simulink model "model_min_mine"  (R2018a)
settings: Solver=ode45  StartTime=0.0  StopTime=20  RelTol=1e-3
(part 3 of 10)

== system model_min_mine/5 систем підйому/1/7-періодні/7-ми періодна криволінійна ==
  note: затримка на
      |  (t1+t1/)
  note: затримка на
      |  (t1+ t2 + t3)
  note: затримка на
      |  (t1+ t2 +t3 + t4 + t4/)
  (t-2) : Saturate  UpperLimit=3.5  LowerLimit=0
  (t-4) : Saturate  UpperLimit=3.5  LowerLimit=0
  (t-5) : Saturate  LowerLimit=0
  (t1) : Saturate  LowerLimit=0
  Clock1 : Clock
      settings: Decimation=14
  Constant : Constant  Value=2
  Divide : Product  Inputs=/
  Integrator : Integrator
  Product3 : Product  SaturateOnIntegerOverflow=on  OutDataTypeStr=Inherit: Same as first input
  Product5 : Product  SaturateOnIntegerOverflow=on  OutDataTypeStr=Inherit: Same as first input
  Product6 : Product  SaturateOnIntegerOverflow=on  OutDataTypeStr=Inherit: Same as first input
  Scope1 : Scope  NumInputPorts=2
  Scope{3..5,7..9} (6 alike) : Scope
  Scope6 : Scope  NumInputPorts=3
  Subsystem : Subsystem
  Subsystem3 : Subsystem
  Subsystem6 : Subsystem
  Sum1 : Sum  Inputs=|++++  SaturateOnIntegerOverflow=on
  Sum2 : Sum  Inputs=|++++  SaturateOnIntegerOverflow=on
  t1 : DeadZone  LowerValue=0  UpperValue=12  SaturateOnIntegerOverflow=on
  t2 : DeadZone  LowerValue=0  UpperValue=1  SaturateOnIntegerOverflow=on
  t5 : DeadZone  LowerValue=0  UpperValue=8  SaturateOnIntegerOverflow=on
  Допоміжний : Subsystem
  Допоміжний1 : Subsystem
  пакет1 : Subsystem
  пакет2 : Subsystem
  постійні : Subsystem
  Out1 : Outport
  Out2 : Outport  Port=2
  Out3 : Outport  Port=3
  wires:
  t2/1 -> (t-2)/1
  Clock1/1 -> t2/1, t5/1, t1/1, Subsystem6/2(t), Subsystem3/1(t1), (t1)/1, Допоміжний/2(t)
  постійні/5(Out5) -> Subsystem/1(t1)
  постійні/1(Out1) -> Product6/2, Subsystem/3(a1)
  (t-2)/1 -> пакет1/2(t)
  постійні/6(Out6) -> пакет1/1(ti)
  постійні/2(Out2) -> пакет1/3(a)
  t5/1 -> (t-4)/1
  (t-4)/1 -> Допоміжний1/2(t), пакет2/2(t)
  t1/1 -> (t-5)/1
  (t-5)/1 -> Product3/1
  постійні/3(Out3) -> пакет2/3(a)
  постійні/4(Out4) -> Subsystem3/3(a1), Product3/2
  Subsystem6/1(Out1) -> Out1/1, Scope1/1
  Product6/1 -> Sum1/1
  Sum1/1 -> Scope3/1, Out2/1, Scope6/2, Scope1/2, Integrator/1
  Subsystem/1(Out1) -> Sum2/2
  (t1)/1 -> Product6/1, Subsystem/2(t)
  Sum2/1 -> Subsystem6/3(a), Scope7/1
  постійні/9(Out9) -> Subsystem6/1(Сума t)
  Product3/1 -> Sum1/4
  Subsystem3/1(Out1) -> Scope9/1, Sum2/4, Scope6/3
  пакет1/1(Out1) -> Допоміжний/3(a1), Scope8/1
  Допоміжний/1(Out1) -> Sum2/1, Scope5/1
  пакет2/1(Out1) -> Допоміжний1/3(a1)
  Допоміжний1/1(Out1) -> Sum2/3, Scope6/1
  постійні/7(Out7) -> Допоміжний1/1(t1), пакет2/1(ti)
  постійні/8(Out8) -> Subsystem3/2(t)
  постійні/11(Out11) -> Допоміжний/1(t1)
  пакет1/2(Out2) -> Sum1/2
  пакет2/2(Out2) -> Sum1/3
  Integrator/1 -> Product5/2
  Product5/1 -> Scope4/1, Out3/1
  Divide/1 -> Product5/1
  Constant/1 -> Divide/1

== system model_min_mine/5 систем підйому/1/7-періодні/7-ми періодна пр ==
  note: затримка на
      |  (t1+t1/)
  note: затримка на
      |  (t1/+t1+ t2 + t3)
  note: затримка на
      |  (t1+ t2 +t3 + t4 + t4/)
  (t-2) : Saturate  UpperLimit=3.5  LowerLimit=0
  (t-4) : Saturate  UpperLimit=3.5  LowerLimit=0
  (t-5) : Saturate  LowerLimit=0
  (t1) : Saturate  LowerLimit=0
  Clock1 : Clock
      settings: Decimation=17
  Constant : Constant  Value=2
  Divide : Product  Inputs=/
  Integrator : Integrator
  Product{2..6} (5 alike) : Product  SaturateOnIntegerOverflow=on  OutDataTypeStr=Inherit: Same as first input
  Scope1 : Scope  NumInputPorts=2
  Scope{2..3,5,7..9} (6 alike) : Scope
  Scope6 : Scope  NumInputPorts=3
  Subsystem : Subsystem
  Subsystem1 : Subsystem
  Subsystem2 : Subsystem
  Subsystem3 : Subsystem
  Subsystem6 : Subsystem
  Sum1 : Sum  Inputs=|++++  SaturateOnIntegerOverflow=on
  Sum2 : Sum  Inputs=|++++  SaturateOnIntegerOverflow=on
  t1 : DeadZone  LowerValue=0  UpperValue=16  SaturateOnIntegerOverflow=on
  t2 : DeadZone  LowerValue=0  UpperValue=1  SaturateOnIntegerOverflow=on
  t5 : DeadZone  LowerValue=0  UpperValue=12  SaturateOnIntegerOverflow=on
  Допоміжний : Subsystem
  Допоміжний1 : Subsystem
  постійні : Subsystem
  Out1 : Outport
  Out2 : Outport  Port=2
  Out3 : Outport  Port=3
  wires:
  t2/1 -> (t-2)/1
  Clock1/1 -> t2/1, t5/1, t1/1, Subsystem6/2(t), Subsystem3/1(t1), Subsystem2/1(t1), (t1)/1, Допоміжний/2(t)
  постійні/5(Out5) -> Subsystem/1(t1)
  постійні/1(Out1) -> Product6/2, Subsystem/3(a1)
  (t-2)/1 -> Product4/1, Subsystem1/2(t)
  постійні/6(Out6) -> Subsystem1/1(t1)
  постійні/2(Out2) -> Product4/2, Subsystem1/3(a1)
  t5/1 -> (t-4)/1
  (t-4)/1 -> Product2/1, Допоміжний1/2(t)
  t1/1 -> (t-5)/1
  (t-5)/1 -> Product3/1
  постійні/3(Out3) -> Subsystem2/3(a1), Product2/2
  постійні/4(Out4) -> Subsystem3/3(a1), Product3/2
  Subsystem6/1(Out1) -> Out1/1, Scope1/1
  Product4/1 -> Sum1/2
  Product6/1 -> Sum1/1
  Sum1/1 -> Scope3/1, Out2/1, Scope6/2, Scope1/2, Integrator/1
  Subsystem/1(Out1) -> Sum2/2
  (t1)/1 -> Product6/1, Subsystem/2(t)
  Sum2/1 -> Subsystem6/3(a), Scope7/1
  постійні/9(Out9) -> Subsystem6/1(Сума t)
  Product2/1 -> Sum1/3
  Product3/1 -> Sum1/4
  Subsystem3/1(Out1) -> Scope9/1, Sum2/4, Scope6/3
  Subsystem1/1(Out1) -> Допоміжний/3(a1), Scope8/1
  Допоміжний/1(Out1) -> Sum2/1, Scope5/1
  постійні/10(Out10) -> Subsystem2/2(t)
  Subsystem2/1(Out1) -> Допоміжний1/3(a1)
  Допоміжний1/1(Out1) -> Sum2/3, Scope6/1
  постійні/7(Out7) -> Допоміжний1/1(t1)
  постійні/8(Out8) -> Subsystem3/2(t)
  постійні/11(Out11) -> Допоміжний/1(t1)
  Integrator/1 -> Product5/2
  Product5/1 -> Scope2/1, Out3/1
  Divide/1 -> Product5/1
  Constant/1 -> Divide/1

== system model_min_mine/5 систем підйому/2/3-періодні/Криволінійна-3 ==
  (t1) : Saturate  UpperLimit=1.15  LowerLimit=0
  (t1+ t2) : DeadZone  LowerValue=0  UpperValue=3.15  SaturateOnIntegerOverflow=on
  Clock1 : Clock
  Constant : Constant  Value=2
  Constant1 : Constant
  Divide : Product  Inputs=/
  Integrator : Integrator
  Product5 : Product  SaturateOnIntegerOverflow=on  OutDataTypeStr=Inherit: Same as first input
  Scope2 : Scope
  Sum1 : Sum  Inputs=|+-  SaturateOnIntegerOverflow=on
  Sum8 : Sum  Inputs=|++  SaturateOnIntegerOverflow=on
  Sum9 : Sum  Inputs=|++  SaturateOnIntegerOverflow=on
  Switch2 : Switch  Criteria=u2 ~= 0  RndMeth=Zero  SaturateOnIntegerOverflow=on
  T-Загальний час циклу,с : Constant  Value=4.3
  V : Scope
  a : Scope
  t3 : Saturate  UpperLimit=1.15  LowerLimit=0
  Генераці1 : Subsystem  TreatAsAtomicUnit=on
  пакет2 : Subsystem
  пакет3 : Subsystem
  постійні : Subsystem
  Out1 : Outport
  Out2 : Outport  Port=2
  Out3 : Outport  Port=3
  wires:
  (t1+ t2)/1 -> t3/1
  Clock1/1 -> (t1)/1, (t1+ t2)/1, Sum1/2
  T-Загальний час циклу,с/1 -> Sum1/1
  Constant1/1 -> Генераці1/1(In1)
  Sum1/1 -> Генераці1/Trigger
  Генераці1/1(Out1) -> Switch2/2
  пакет3/1(Out1) -> Sum8/2
  пакет3/2(Out2) -> Sum9/2
  пакет2/1(Out1) -> Sum8/1
  Sum8/1 -> Switch2/3, a/1
  Switch2/1 -> Out1/1
  Sum9/1 -> Out2/1, V/1, Integrator/1
  пакет2/2(Out2) -> Sum9/1
  постійні/1(Out1) -> пакет2/3(a)
  постійні/2(Out2) -> пакет3/3(a)
  постійні/4(Out4) -> пакет3/1(ti)
  постійні/3(Out3) -> пакет2/1(ti)
  (t1)/1 -> пакет2/2(t)
  t3/1 -> пакет3/2(t)
  Integrator/1 -> Product5/2
  Product5/1 -> Scope2/1, Out3/1
  Divide/1 -> Product5/1
  Constant/1 -> Divide/1

== system model_min_mine/5 систем підйому/2/3-періодні/Пр ==
  note: (t1+t2)
  (t1) : Saturate  UpperLimit=1.15  LowerLimit=0
  Clock1 : Clock
  Constant : Constant  Value=2
  Constant1 : Constant
  Constant2 : Constant
  Constant5 : Constant
  Divide : Product  Inputs=/
  Integrator : Integrator
  Product2 : Product  SaturateOnIntegerOverflow=on  OutDataTypeStr=Inherit: Same as first input
  Product5 : Product  SaturateOnIntegerOverflow=on  OutDataTypeStr=Inherit: Same as first input
  Product6 : Product  SaturateOnIntegerOverflow=on  OutDataTypeStr=Inherit: Same as first input
  Scope2 : Scope
  Sum1 : Sum  Inputs=|+-  SaturateOnIntegerOverflow=on
  Sum2 : Sum  Inputs=|+-  SaturateOnIntegerOverflow=on
  Sum4 : Sum  Inputs=|+-  SaturateOnIntegerOverflow=on
  Sum8 : Sum  Inputs=|++  SaturateOnIntegerOverflow=on
  Sum9 : Sum  Inputs=|++  SaturateOnIntegerOverflow=on
  Switch1 : Switch  Criteria=u2 ~= 0  RndMeth=Zero  SaturateOnIntegerOverflow=on
  Switch2 : Switch  Criteria=u2 ~= 0  RndMeth=Zero  SaturateOnIntegerOverflow=on
  Switch3 : Switch  Criteria=u2 ~= 0  RndMeth=Zero  SaturateOnIntegerOverflow=on
  T-Загальний час циклу,с : Constant  Value=4.3
  V : Scope
  V1 : Scope
  ogr : Saturate  UpperLimit=100  LowerLimit=0
  t2 : DeadZone  LowerValue=0  UpperValue=3.15  SaturateOnIntegerOverflow=on
  t3 : Saturate  UpperLimit=1.15  LowerLimit=0
  Генераці : Subsystem  TreatAsAtomicUnit=on
  Генераці1 : Subsystem  TreatAsAtomicUnit=on
  Генераці2 : Subsystem  TreatAsAtomicUnit=on
  постійні : Subsystem
  Out1 : Outport
  Out2 : Outport  Port=2
  Out3 : Outport  Port=3
  wires:
  постійні/1(Out1) -> Product6/1, Switch1/3
  t2/1 -> t3/1
  t3/1 -> Product2/2
  Clock1/1 -> (t1)/1, t2/1, Sum2/1, Sum1/2
  (t1)/1 -> Product6/2, Sum4/2
  Product6/1 -> Sum9/1
  постійні/2(Out2) -> Product2/1, Switch2/1
  Product2/1 -> Sum9/2
  Sum9/1 -> ogr/1, V/1, Integrator/1
  Constant5/1 -> Генераці/1(In1)
  Sum4/1 -> Генераці/Trigger
  Генераці/1(Out1) -> Switch1/2
  Switch1/1 -> Sum8/1
  постійні/4(Out4) -> Sum4/1
  Constant1/1 -> Генераці1/1(In1)
  Sum1/1 -> Генераці1/Trigger
  Генераці1/1(Out1) -> Switch2/2
  Switch2/1 -> Sum8/2
  ogr/1 -> Out2/1
  Constant2/1 -> Генераці2/1(In1)
  Генераці2/1(Out1) -> Switch3/2
  Sum2/1 -> Генераці2/Trigger
  Sum8/1 -> Switch3/3
  Switch3/1 -> Out1/1, V1/1
  постійні/5(Out5) -> Sum1/1
  T-Загальний час циклу,с/1 -> Sum2/2
  Integrator/1 -> Product5/2
  Product5/1 -> Scope2/1, Out3/1
  Divide/1 -> Product5/1
  Constant/1 -> Divide/1

== system model_min_mine/5 систем підйому/2/4-періодна /Генераці ==
  In1 : Inport
  Trigger : TriggerPort  TriggerType=either  VariantControl=(inherit)  ShowOutputPort=on
  Out1 : Outport
  wires:
  In1/1 -> Out1/1

== system model_min_mine/5 систем підйому/2/4-періодна /Генераці1 ==
  In1 : Inport
  Trigger : TriggerPort  TriggerType=either  VariantControl=(inherit)  ShowOutputPort=on
  Out1 : Outport
  wires:
  In1/1 -> Out1/1

== system model_min_mine/5 систем підйому/2/4-періодна /Генераці2 ==
  In1 : Inport
  Trigger : TriggerPort  TriggerType=either  VariantControl=(inherit)  ShowOutputPort=on
  Out1 : Outport
  wires:
  In1/1 -> Out1/1

== system model_min_mine/5 систем підйому/2/4-періодна /Генераці3 ==
  In1 : Inport
  Trigger : TriggerPort  TriggerType=either  VariantControl=(inherit)  ShowOutputPort=on
  Out1 : Outport
  wires:
  In1/1 -> Out1/1

== system model_min_mine/5 систем підйому/2/4-періодна /постійні ==
  (t1) : Constant  Value=1.15
  (t3) : Constant  Value=2
  (t4) : Constant
  T : Constant  Value=7.15
  a1 : Constant  Value=0.5
  a3 : Constant  Value=-1
  a4 : Constant  Value=-0.95
  Out1 : Outport
  Out2 : Outport  Port=2
  Out6 : Outport  Port=3
  Out3 : Outport  Port=4
  Out4 : Outport  Port=5
  Out5 : Outport  Port=6
  Out7 : Outport  Port=7
  wires:
  a1/1 -> Out1/1
  a3/1 -> Out2/1
  (t3)/1 -> Out3/1
  (t1)/1 -> Out4/1
  (t4)/1 -> Out5/1
  a4/1 -> Out6/1
  T/1 -> Out7/1

== system model_min_mine/5 систем підйому/2/5-періодні/криво ==
  note: затримка на
      |  (t1)
  note: затримка на
      |  (t1+ t2 + t3)
  note: затримка на
      |  (t1+ t2 +t3 +t4)
  (t-2) : Saturate  UpperLimit=3.5  LowerLimit=0
  (t-4) : Saturate  UpperLimit=3.5  LowerLimit=0
  (t-5) : Saturate  LowerLimit=0
  (t1) : Saturate  LowerLimit=0
  Clock1 : Clock
      settings: Decimation=14
  Constant : Constant  Value=2
  Divide : Product  Inputs=/
  Integrator : Integrator
  Product{2..6} (5 alike) : Product  SaturateOnIntegerOverflow=on  OutDataTypeStr=Inherit: Same as first input
  Scope{1..3,5..7,9} (7 alike) : Scope
  Subsystem : Subsystem
  Subsystem1 : Subsystem
  Subsystem2 : Subsystem
  Subsystem3 : Subsystem
  Subsystem6 : Subsystem
  Sum1 : Sum  Inputs=|++++  SaturateOnIntegerOverflow=on
  Sum2 : Sum  Inputs=|++++  SaturateOnIntegerOverflow=on
  t1 : DeadZone  LowerValue=0  UpperValue=11.5  SaturateOnIntegerOverflow=on
  t2 : DeadZone  LowerValue=0  SaturateOnIntegerOverflow=on
  t5 : DeadZone  LowerValue=0  UpperValue=8  SaturateOnIntegerOverflow=on
  Допоміжний : Subsystem
  Допоміжний1 : Subsystem
  постійні : Subsystem
  Out1 : Outport
  Out2 : Outport  Port=2
  Out3 : Outport  Port=3
  wires:
  t2/1 -> (t-2)/1
  Clock1/1 -> t2/1, t5/1, t1/1, Subsystem6/2(t), Subsystem3/1(t1), Subsystem2/1(t1), (t1)/1
  постійні/5(Out5) -> Subsystem/1(t1)
  постійні/1(Out1) -> Product6/2, Subsystem/3(a1)
  (t-2)/1 -> Product4/1, Subsystem1/2(t)
  постійні/6(Out6) -> Subsystem1/1(t1)
  постійні/2(Out2) -> Product4/2, Subsystem1/3(a1)
  t5/1 -> (t-4)/1
  (t-4)/1 -> Product2/1, Допоміжний1/2(t)
  t1/1 -> (t-5)/1
  (t-5)/1 -> Product3/1
  постійні/3(Out3) -> Subsystem2/3(a1), Product2/2
  постійні/4(Out4) -> Subsystem3/3(a1), Product3/2
  Subsystem6/1(Out1) -> Out1/1, Scope1/1
  Product4/1 -> Sum1/2
  Product6/1 -> Sum1/1
  Sum1/1 -> Scope3/1, Out2/1, Integrator/1
  Subsystem/1(Out1) -> Допоміжний/1(t1), Scope5/1, Sum2/2
  (t1)/1 -> Product6/1, Subsystem/2(t), Допоміжний/2(t)
  Sum2/1 -> Subsystem6/3(a), Scope7/1
  постійні/9(Out9) -> Subsystem6/1(Сума t)
  Product2/1 -> Sum1/3, Scope6/1
  Product3/1 -> Sum1/4
  Subsystem3/1(Out1) -> Scope9/1, Sum2/4
  Subsystem1/1(Out1) -> Допоміжний/3(a1)
  Допоміжний/1(Out1) -> Sum2/1
  постійні/10(Out10) -> Subsystem2/2(t)
  Subsystem2/1(Out1) -> Допоміжний1/3(a1)
  Допоміжний1/1(Out1) -> Sum2/3
  постійні/7(Out7) -> Допоміжний1/1(t1)
  постійні/8(Out8) -> Subsystem3/2(t)
  Integrator/1 -> Product5/2
  Product5/1 -> Scope2/1, Out3/1
  Divide/1 -> Product5/1
  Constant/1 -> Divide/1

== system model_min_mine/5 систем підйому/2/5-періодні/пр ==
  note: затримка на
      |  (t1)
  note: затримка на
      |  (t1+ t2)
  note: затримка на
      |  (t1+ t2 +t3 +t4)
  note: затримка на
      |  (t1+ t2 +t3 +t4 +t5)
  note: затримка на
      |  (t1+ t2 +t3 +t4 +t5 + t6)
  (t-2) : Saturate  UpperLimit=3.5  LowerLimit=0
  (t-3) : Saturate  LowerLimit=0
  (t-5) : Saturate  LowerLimit=0
  (t-6) : Saturate  UpperLimit=3.5  LowerLimit=0
  (t-7) : Saturate  LowerLimit=0
  (t1) : Saturate  LowerLimit=0
  Clock1 : Clock
      settings: Decimation=14
  Constant : Constant  Value=2
  Divide : Product  Inputs=/
  Integrator : Integrator
  Product{1,4..7} (5 alike) : Product  SaturateOnIntegerOverflow=on  OutDataTypeStr=Inherit: Same as first input
  Scope{1..3,5} (4 alike) : Scope
  Subsystem : Subsystem
  Subsystem1 : Subsystem
  Subsystem4 : Subsystem
  Subsystem5 : Subsystem
  Subsystem6 : Subsystem
  Sum1 : Sum  Inputs=|++++++  SaturateOnIntegerOverflow=on
  Sum2 : Sum  Inputs=|++++  SaturateOnIntegerOverflow=on
  Sum3 : Sum  Inputs=-  SaturateOnIntegerOverflow=on
  t1 : DeadZone  LowerValue=0  UpperValue=7.5  SaturateOnIntegerOverflow=on
  t2 : DeadZone  LowerValue=0  SaturateOnIntegerOverflow=on
  t3 : DeadZone  LowerValue=0  UpperValue=8  SaturateOnIntegerOverflow=on
  t4 : DeadZone  LowerValue=0  UpperValue=11.5  SaturateOnIntegerOverflow=on
  t5 : DeadZone  LowerValue=0  UpperValue=4  SaturateOnIntegerOverflow=on
  Допоміжний : Subsystem
  Допоміжний -1 : Subsystem
  Допоміжний -2 : Subsystem
  Допоміжний -3 : Subsystem
  Допоміжний -4 : Subsystem
  пакет1 : Subsystem
  пакет2 : Subsystem
  постійні : Subsystem
  Out1 : Outport
  Out2 : Outport  Port=2
  Out3 : Outport  Port=3
  wires:
  t2/1 -> (t-2)/1
  Clock1/1 -> t2/1, t5/1, t1/1, t3/1, t4/1, Subsystem6/2(t), (t1)/1
  постійні/7(Out7) -> Subsystem/1(t1)
  постійні/1(Out1) -> Product6/2, Subsystem/3(a1)
  (t-2)/1 -> Product4/1, Subsystem1/2(t), Допоміжний -1/2(t)
  постійні/8(Out8) -> Subsystem1/1(t1)
  постійні/2(Out2) -> Product4/2, Subsystem1/3(a1)
  t5/1 -> (t-3)/1
  (t-3)/1 -> пакет1/2(t), Допоміжний -2/2(t)
  t1/1 -> (t-5)/1
  (t-5)/1 -> пакет2/2(t), Допоміжний -3/2(t)
  постійні/9(Out9) -> пакет1/1(ti)
  постійні/11(Out11) -> пакет2/1(ti)
  постійні/3(Out3) -> пакет1/3(a)
  постійні/4(Out4) -> пакет2/3(a)
  t3/1 -> (t-6)/1
  (t-6)/1 -> Product5/1, Subsystem4/2(t), Допоміжний -4/2(t)
  постійні/12(Out12) -> Subsystem4/1(ti)
  постійні/5(Out5) -> Subsystem4/3(a), Product5/2
  t4/1 -> (t-7)/1
  (t-7)/1 -> Subsystem5/2(t), Product7/1
  постійні/13(Out13) -> Subsystem5/1(ti)
  постійні/6(Out6) -> Product7/2, Subsystem5/3(a)
  постійні/10(Out10) -> Subsystem6/1(Сума t)
  Subsystem6/1(Out1) -> Out1/1, Scope1/1
  Product4/1 -> Sum1/2
  Product6/1 -> Sum1/1
  пакет1/2(Out2) -> Sum1/3
  пакет2/2(Out2) -> Sum1/4
  Product5/1 -> Sum1/5
  Product7/1 -> Sum1/6
  Sum1/1 -> Scope3/1, Out2/1, Integrator/1
  Subsystem/1(Out1) -> Допоміжний/1(t1), Sum2/2, Scope5/1
  (t1)/1 -> Product6/1, Subsystem/2(t), Допоміжний/2(t)
  Subsystem1/1(Out1) -> Допоміжний/3(a1)
  Допоміжний/1(Out1) -> Допоміжний -1/1(t1)
  пакет1/1(Out1) -> Допоміжний -1/3(a1)
  Допоміжний -1/1(Out1) -> Допоміжний -2/1(t1), Sum2/1
  пакет2/1(Out1) -> Допоміжний -2/3(a1)
  Допоміжний -2/1(Out1) -> Допоміжний -3/1(t1), Sum2/3
  Subsystem4/1(Out1) -> Допоміжний -3/3(a1)
  Допоміжний -3/1(Out1) -> Допоміжний -4/1(t1)
  Subsystem5/1(Out1) -> Допоміжний -4/3(a1)
  Sum2/1 -> Subsystem6/3(a)
  Допоміжний -4/1(Out1) -> Sum3/1
  Sum3/1 -> Sum2/4
  Integrator/1 -> Product1/2
  Product1/1 -> Scope2/1, Out3/1
  Divide/1 -> Product1/1
  Constant/1 -> Divide/1

== system model_min_mine/5 систем підйому/2/6-періодні/6-ти періодна криволінійна ==
  note: затримка на
      |  (t1)
  note: затримка на
      |  (t1+ t2 + t3)
  note: затримка на
      |  (t1+ t2 +t3 +t4 +t4/)
  (t-2) : Saturate  UpperLimit=3.5  LowerLimit=0
  (t-4) : Saturate  UpperLimit=3.5  LowerLimit=0
  (t-5) : Saturate  LowerLimit=0
  (t1) : Saturate  LowerLimit=0
  Clock1 : Clock
      settings: Decimation=14
  Constant : Constant  Value=2
  Divide : Product  Inputs=/
  Integrator : Integrator
  Product3 : Product  SaturateOnIntegerOverflow=on  OutDataTypeStr=Inherit: Same as first input
  Product5 : Product  SaturateOnIntegerOverflow=on  OutDataTypeStr=Inherit: Same as first input
  Product6 : Product  SaturateOnIntegerOverflow=on  OutDataTypeStr=Inherit: Same as first input
  Scope{1..3,5,7,9} (6 alike) : Scope
  Scope6 : Scope  NumInputPorts=3
  Subsystem : Subsystem
  Subsystem3 : Subsystem
  Subsystem6 : Subsystem
  Sum1 : Sum  Inputs=|++++  SaturateOnIntegerOverflow=on
  Sum2 : Sum  Inputs=|++++  SaturateOnIntegerOverflow=on
  t1 : DeadZone  LowerValue=0  UpperValue=12  SaturateOnIntegerOverflow=on
  t2 : DeadZone  LowerValue=0  SaturateOnIntegerOverflow=on
  t5 : DeadZone  LowerValue=0  UpperValue=8  SaturateOnIntegerOverflow=on
  Допоміжний : Subsystem
  Допоміжний1 : Subsystem
  пакет1 : Subsystem
  пакет2 : Subsystem
  постійні : Subsystem
  Out1 : Outport
  Out2 : Outport  Port=2
  Out3 : Outport  Port=3
  wires:
  t2/1 -> (t-2)/1
  Clock1/1 -> (t1)/1, t2/1, t5/1, t1/1, Subsystem6/2(t), Subsystem3/1(t1)
  постійні/5(Out5) -> Subsystem/1(t1)
  постійні/1(Out1) -> Product6/2, Subsystem/3(a1)
  (t-2)/1 -> пакет1/2(t)
  постійні/6(Out6) -> пакет1/1(ti)
  постійні/2(Out2) -> пакет1/3(a)
  t5/1 -> (t-4)/1
  (t-4)/1 -> Допоміжний1/2(t), пакет2/2(t)
  t1/1 -> (t-5)/1
  (t-5)/1 -> Product3/1
  постійні/3(Out3) -> пакет2/3(a)
  постійні/4(Out4) -> Subsystem3/3(a1), Product3/2
  Subsystem6/1(Out1) -> Out1/1, Scope1/1
  Product6/1 -> Sum1/1
  Sum1/1 -> Scope3/1, Out2/1, Scope6/2, Integrator/1
  Subsystem/1(Out1) -> Допоміжний/1(t1), Scope5/1, Sum2/2
  (t1)/1 -> Product6/1, Subsystem/2(t), Допоміжний/2(t)
  Sum2/1 -> Subsystem6/3(a), Scope7/1
  постійні/9(Out9) -> Subsystem6/1(Сума t)
  Product3/1 -> Sum1/4
  Subsystem3/1(Out1) -> Scope9/1, Sum2/4, Scope6/3
  пакет1/1(Out1) -> Допоміжний/3(a1)
  Допоміжний/1(Out1) -> Sum2/1
  пакет2/1(Out1) -> Допоміжний1/3(a1)
  Допоміжний1/1(Out1) -> Sum2/3, Scope6/1
  постійні/7(Out7) -> Допоміжний1/1(t1), пакет2/1(ti)
  постійні/8(Out8) -> Subsystem3/2(t)
  пакет1/2(Out2) -> Sum1/2
  пакет2/2(Out2) -> Sum1/3
  Integrator/1 -> Product5/2
  Product5/1 -> Scope2/1, Out3/1
  Divide/1 -> Product5/1
  Constant/1 -> Divide/1

== system model_min_mine/5 систем підйому/2/6-періодні/6-ти періодна пр ==
  note: затримка на
      |  (t1)
  note: затримка на
      |  (t1+ t2 + t3)
  note: затримка на
      |  (t1+ t2 +t3 +t4 +t4/)
  (t-2) : Saturate  UpperLimit=3.5  LowerLimit=0
  (t-4) : Saturate  UpperLimit=3.5  LowerLimit=0
  (t-5) : Saturate  LowerLimit=0
  (t1) : Saturate  LowerLimit=0
  Clock1 : Clock
      settings: Decimation=14
  Constant : Constant  Value=2
  Divide : Product  Inputs=/
  Integrator : Integrator
  Product{2..6} (5 alike) : Product  SaturateOnIntegerOverflow=on  OutDataTypeStr=Inherit: Same as first input
  Scope{1..3,5,7,9} (6 alike) : Scope
  Scope6 : Scope  NumInputPorts=3
  Subsystem : Subsystem
  Subsystem1 : Subsystem
  Subsystem2 : Subsystem
  Subsystem3 : Subsystem
  Subsystem6 : Subsystem
  Sum1 : Sum  Inputs=|++++  SaturateOnIntegerOverflow=on
  Sum2 : Sum  Inputs=|++++  SaturateOnIntegerOverflow=on
  t1 : DeadZone  LowerValue=0  UpperValue=12  SaturateOnIntegerOverflow=on
  t2 : DeadZone  LowerValue=0  SaturateOnIntegerOverflow=on
  t5 : DeadZone  LowerValue=0  UpperValue=8  SaturateOnIntegerOverflow=on
  Допоміжний : Subsystem
  Допоміжний1 : Subsystem
  постійні : Subsystem
  Out1 : Outport
  Out2 : Outport  Port=2
  Out3 : Outport  Port=3
  wires:
  t2/1 -> (t-2)/1
  Clock1/1 -> t2/1, t5/1, t1/1, Subsystem6/2(t), Subsystem3/1(t1), Subsystem2/1(t1), (t1)/1
  постійні/5(Out5) -> Subsystem/1(t1)
  постійні/1(Out1) -> Product6/2, Subsystem/3(a1)
  (t-2)/1 -> Product4/1, Subsystem1/2(t)
  постійні/6(Out6) -> Subsystem1/1(t1)
  постійні/2(Out2) -> Product4/2, Subsystem1/3(a1)
  t5/1 -> (t-4)/1
  (t-4)/1 -> Product2/1, Допоміжний1/2(t)
  t1/1 -> (t-5)/1
  (t-5)/1 -> Product3/1
  постійні/3(Out3) -> Subsystem2/3(a1), Product2/2
  постійні/4(Out4) -> Subsystem3/3(a1), Product3/2
  Subsystem6/1(Out1) -> Out1/1, Scope1/1
  Product4/1 -> Sum1/2
  Product6/1 -> Sum1/1
  Sum1/1 -> Scope3/1, Out2/1, Scope6/2, Integrator/1
  Subsystem/1(Out1) -> Допоміжний/1(t1), Scope5/1, Sum2/2
  (t1)/1 -> Product6/1, Subsystem/2(t), Допоміжний/2(t)
  Sum2/1 -> Subsystem6/3(a), Scope7/1
  постійні/9(Out9) -> Subsystem6/1(Сума t)
  Product2/1 -> Sum1/3
  Product3/1 -> Sum1/4
  Subsystem3/1(Out1) -> Scope9/1, Sum2/4, Scope6/3
  Subsystem1/1(Out1) -> Допоміжний/3(a1)
  Допоміжний/1(Out1) -> Sum2/1
  постійні/10(Out10) -> Subsystem2/2(t)
  Subsystem2/1(Out1) -> Допоміжний1/3(a1)
  Допоміжний1/1(Out1) -> Sum2/3, Scope6/1
  постійні/7(Out7) -> Допоміжний1/1(t1)
  постійні/8(Out8) -> Subsystem3/2(t)
  Integrator/1 -> Product5/2
  Product5/1 -> Scope2/1, Out3/1
  Divide/1 -> Product5/1
  Constant/1 -> Divide/1

== system model_min_mine/5 систем підйому/2/7-періодні/7-ми періодна криволінійна ==
  note: затримка на
      |  (t1+t1/)
  note: затримка на
      |  (t1+ t2 + t3)
  note: затримка на
      |  (t1+ t2 +t3 + t4 + t4/)
  (t-2) : Saturate  UpperLimit=3.5  LowerLimit=0
  (t-4) : Saturate  UpperLimit=3.5  LowerLimit=0
  (t-5) : Saturate  LowerLimit=0
  (t1) : Saturate  LowerLimit=0
  Clock1 : Clock
      settings: Decimation=14
  Constant : Constant  Value=2
  Divide : Product  Inputs=/
  Integrator : Integrator
  Product3 : Product  SaturateOnIntegerOverflow=on  OutDataTypeStr=Inherit: Same as first input
  Product5 : Product  SaturateOnIntegerOverflow=on  OutDataTypeStr=Inherit: Same as first input
  Product6 : Product  SaturateOnIntegerOverflow=on  OutDataTypeStr=Inherit: Same as first input
  Scope1 : Scope  NumInputPorts=2
  Scope{3..5,7..9} (6 alike) : Scope
  Scope6 : Scope  NumInputPorts=3
  Subsystem : Subsystem
  Subsystem3 : Subsystem
  Subsystem6 : Subsystem
  Sum1 : Sum  Inputs=|++++  SaturateOnIntegerOverflow=on
  Sum2 : Sum  Inputs=|++++  SaturateOnIntegerOverflow=on
  t1 : DeadZone  LowerValue=0  UpperValue=12  SaturateOnIntegerOverflow=on
  t2 : DeadZone  LowerValue=0  UpperValue=1  SaturateOnIntegerOverflow=on
  t5 : DeadZone  LowerValue=0  UpperValue=8  SaturateOnIntegerOverflow=on
  Допоміжний : Subsystem
  Допоміжний1 : Subsystem
  пакет1 : Subsystem
  пакет2 : Subsystem
  постійні : Subsystem
  Out1 : Outport
  Out2 : Outport  Port=2
  Out3 : Outport  Port=3
  wires:
  t2/1 -> (t-2)/1
  Clock1/1 -> t2/1, t5/1, t1/1, Subsystem6/2(t), Subsystem3/1(t1), (t1)/1, Допоміжний/2(t)
  постійні/5(Out5) -> Subsystem/1(t1)
  постійні/1(Out1) -> Product6/2, Subsystem/3(a1)
  (t-2)/1 -> пакет1/2(t)
  постійні/6(Out6) -> пакет1/1(ti)
  постійні/2(Out2) -> пакет1/3(a)
  t5/1 -> (t-4)/1
  (t-4)/1 -> Допоміжний1/2(t), пакет2/2(t)
  t1/1 -> (t-5)/1
  (t-5)/1 -> Product3/1
  постійні/3(Out3) -> пакет2/3(a)
  постійні/4(Out4) -> Subsystem3/3(a1), Product3/2
  Subsystem6/1(Out1) -> Out1/1, Scope1/1
  Product6/1 -> Sum1/1
  Sum1/1 -> Scope3/1, Out2/1, Scope6/2, Scope1/2, Integrator/1
  Subsystem/1(Out1) -> Sum2/2
  (t1)/1 -> Product6/1, Subsystem/2(t)
  Sum2/1 -> Subsystem6/3(a), Scope7/1
  постійні/9(Out9) -> Subsystem6/1(Сума t)
  Product3/1 -> Sum1/4
  Subsystem3/1(Out1) -> Scope9/1, Sum2/4, Scope6/3
  пакет1/1(Out1) -> Допоміжний/3(a1), Scope8/1
  Допоміжний/1(Out1) -> Sum2/1, Scope5/1
  пакет2/1(Out1) -> Допоміжний1/3(a1)
  Допоміжний1/1(Out1) -> Sum2/3, Scope6/1
  постійні/7(Out7) -> Допоміжний1/1(t1), пакет2/1(ti)
  постійні/8(Out8) -> Subsystem3/2(t)
  постійні/11(Out11) -> Допоміжний/1(t1)
  пакет1/2(Out2) -> Sum1/2
  пакет2/2(Out2) -> Sum1/3
  Integrator/1 -> Product5/2
  Product5/1 -> Scope4/1, Out3/1
  Divide/1 -> Product5/1
  Constant/1 -> Divide/1

== system model_min_mine/5 систем підйому/2/7-періодні/7-ми періодна пр ==
  note: затримка на
      |  (t1+t1/)
  note: затримка на
      |  (t1/+t1+ t2 + t3)
  note: затримка на
      |  (t1+ t2 +t3 + t4 + t4/)
  (t-2) : Saturate  UpperLimit=3.5  LowerLimit=0
  (t-4) : Saturate  UpperLimit=3.5  LowerLimit=0
  (t-5) : Saturate  LowerLimit=0
  (t1) : Saturate  LowerLimit=0
  Clock1 : Clock
      settings: Decimation=17
  Constant : Constant  Value=2
  Divide : Product  Inputs=/
  Integrator : Integrator
  Product{2..6} (5 alike) : Product  SaturateOnIntegerOverflow=on  OutDataTypeStr=Inherit: Same as first input
  Scope1 : Scope  NumInputPorts=2
  Scope{2..3,5,7..9} (6 alike) : Scope
  Scope6 : Scope  NumInputPorts=3
  Subsystem : Subsystem
  Subsystem1 : Subsystem
  Subsystem2 : Subsystem
  Subsystem3 : Subsystem
  Subsystem6 : Subsystem
  Sum1 : Sum  Inputs=|++++  SaturateOnIntegerOverflow=on
  Sum2 : Sum  Inputs=|++++  SaturateOnIntegerOverflow=on
  t1 : DeadZone  LowerValue=0  UpperValue=16  SaturateOnIntegerOverflow=on
  t2 : DeadZone  LowerValue=0  UpperValue=1  SaturateOnIntegerOverflow=on
  t5 : DeadZone  LowerValue=0  UpperValue=12  SaturateOnIntegerOverflow=on
  Допоміжний : Subsystem
  Допоміжний1 : Subsystem
  постійні : Subsystem
  Out1 : Outport
  Out2 : Outport  Port=2
  Out3 : Outport  Port=3
  wires:
  t2/1 -> (t-2)/1
  Clock1/1 -> t2/1, t5/1, t1/1, Subsystem6/2(t), Subsystem3/1(t1), Subsystem2/1(t1), (t1)/1, Допоміжний/2(t)
  постійні/5(Out5) -> Subsystem/1(t1)
  постійні/1(Out1) -> Product6/2, Subsystem/3(a1)
  (t-2)/1 -> Product4/1, Subsystem1/2(t)
  постійні/6(Out6) -> Subsystem1/1(t1)
  постійні/2(Out2) -> Product4/2, Subsystem1/3(a1)
  t5/1 -> (t-4)/1
  (t-4)/1 -> Product2/1, Допоміжний1/2(t)
  t1/1 -> (t-5)/1
  (t-5)/1 -> Product3/1
  постійні/3(Out3) -> Subsystem2/3(a1), Product2/2
  постійні/4(Out4) -> Subsystem3/3(a1), Product3/2
  Subsystem6/1(Out1) -> Out1/1, Scope1/1
  Product4/1 -> Sum1/2
  Product6/1 -> Sum1/1
  Sum1/1 -> Scope3/1, Out2/1, Scope6/2, Scope1/2, Integrator/1
  Subsystem/1(Out1) -> Sum2/2
  (t1)/1 -> Product6/1, Subsystem/2(t)
  Sum2/1 -> Subsystem6/3(a), Scope7/1
  постійні/9(Out9) -> Subsystem6/1(Сума t)
  Product2/1 -> Sum1/3
  Product3/1 -> Sum1/4
  Subsystem3/1(Out1) -> Scope9/1, Sum2/4, Scope6/3
  Subsystem1/1(Out1) -> Допоміжний/3(a1), Scope8/1
  Допоміжний/1(Out1) -> Sum2/1, Scope5/1
  постійні/10(Out10) -> Subsystem2/2(t)
  Subsystem2/1(Out1) -> Допоміжний1/3(a1)
  Допоміжний1/1(Out1) -> Sum2/3, Scope6/1
  постійні/7(Out7) -> Допоміжний1/1(t1)
  постійні/8(Out8) -> Subsystem3/2(t)
  постійні/11(Out11) -> Допоміжний/1(t1)
  Integrator/1 -> Product5/2
  Product5/1 -> Scope2/1, Out3/1
  Divide/1 -> Product5/1
  Constant/1 -> Divide/1

== system model_min_mine/5 систем підйому/3/3-періодні/Криволінійна-3 ==
  (t1) : Saturate  UpperLimit=1.15  LowerLimit=0
  (t1+ t2) : DeadZone  LowerValue=0  UpperValue=3.15  SaturateOnIntegerOverflow=on
  Clock1 : Clock
  Constant : Constant  Value=2
  Constant1 : Constant
  Divide : Product  Inputs=/
  Integrator : Integrator
  Product5 : Product  SaturateOnIntegerOverflow=on  OutDataTypeStr=Inherit: Same as first input
  Scope2 : Scope
  Sum1 : Sum  Inputs=|+-  SaturateOnIntegerOverflow=on
  Sum8 : Sum  Inputs=|++  SaturateOnIntegerOverflow=on
  Sum9 : Sum  Inputs=|++  SaturateOnIntegerOverflow=on
  Switch2 : Switch  Criteria=u2 ~= 0  RndMeth=Zero  SaturateOnIntegerOverflow=on
  T-Загальний час циклу,с : Constant  Value=4.3
  V : Scope
  a : Scope
  t3 : Saturate  UpperLimit=1.15  LowerLimit=0
  Генераці1 : Subsystem  TreatAsAtomicUnit=on
  пакет2 : Subsystem
  пакет3 : Subsystem
  постійні : Subsystem
  Out1 : Outport
  Out2 : Outport  Port=2
  Out3 : Outport  Port=3
  wires:
  (t1+ t2)/1 -> t3/1
  Clock1/1 -> (t1)/1, (t1+ t2)/1, Sum1/2
  T-Загальний час циклу,с/1 -> Sum1/1
  Constant1/1 -> Генераці1/1(In1)
  Sum1/1 -> Генераці1/Trigger
  Генераці1/1(Out1) -> Switch2/2
  пакет3/1(Out1) -> Sum8/2
  пакет3/2(Out2) -> Sum9/2
  пакет2/1(Out1) -> Sum8/1
  Sum8/1 -> Switch2/3, a/1
  Switch2/1 -> Out1/1
  Sum9/1 -> Out2/1, V/1, Integrator/1
  пакет2/2(Out2) -> Sum9/1
  постійні/1(Out1) -> пакет2/3(a)
  постійні/2(Out2) -> пакет3/3(a)
  постійні/4(Out4) -> пакет3/1(ti)
  постійні/3(Out3) -> пакет2/1(ti)
  (t1)/1 -> пакет2/2(t)
  t3/1 -> пакет3/2(t)
  Integrator/1 -> Product5/2
  Product5/1 -> Scope2/1, Out3/1
  Divide/1 -> Product5/1
  Constant/1 -> Divide/1

== system model_min_mine/5 систем підйому/3/3-періодні/Пр ==
  note: (t1+t2)
  (t1) : Saturate  UpperLimit=1.15  LowerLimit=0
  Clock1 : Clock
  Constant : Constant  Value=2
  Constant1 : Constant
  Constant2 : Constant
  Constant5 : Constant
  Divide : Product  Inputs=/
  Integrator : Integrator
  Product2 : Product  SaturateOnIntegerOverflow=on  OutDataTypeStr=Inherit: Same as first input
  Product5 : Product  SaturateOnIntegerOverflow=on  OutDataTypeStr=Inherit: Same as first input
  Product6 : Product  SaturateOnIntegerOverflow=on  OutDataTypeStr=Inherit: Same as first input
  Scope2 : Scope
  Sum1 : Sum  Inputs=|+-  SaturateOnIntegerOverflow=on
  Sum2 : Sum  Inputs=|+-  SaturateOnIntegerOverflow=on
  Sum4 : Sum  Inputs=|+-  SaturateOnIntegerOverflow=on
  Sum8 : Sum  Inputs=|++  SaturateOnIntegerOverflow=on
  Sum9 : Sum  Inputs=|++  SaturateOnIntegerOverflow=on
  Switch1 : Switch  Criteria=u2 ~= 0  RndMeth=Zero  SaturateOnIntegerOverflow=on
  Switch2 : Switch  Criteria=u2 ~= 0  RndMeth=Zero  SaturateOnIntegerOverflow=on
  Switch3 : Switch  Criteria=u2 ~= 0  RndMeth=Zero  SaturateOnIntegerOverflow=on
  T-Загальний час циклу,с : Constant  Value=4.3
  V : Scope
  V1 : Scope
  ogr : Saturate  UpperLimit=100  LowerLimit=0
  t2 : DeadZone  LowerValue=0  UpperValue=3.15  SaturateOnIntegerOverflow=on
  t3 : Saturate  UpperLimit=1.15  LowerLimit=0
  Генераці : Subsystem  TreatAsAtomicUnit=on
  Генераці1 : Subsystem  TreatAsAtomicUnit=on
  Генераці2 : Subsystem  TreatAsAtomicUnit=on
  постійні : Subsystem
  Out1 : Outport
  Out2 : Outport  Port=2
  Out3 : Outport  Port=3
  wires:
  постійні/1(Out1) -> Product6/1, Switch1/3
  t2/1 -> t3/1
  t3/1 -> Product2/2
  Clock1/1 -> (t1)/1, t2/1, Sum2/1, Sum1/2
  (t1)/1 -> Product6/2, Sum4/2
  Product6/1 -> Sum9/1
  постійні/2(Out2) -> Product2/1, Switch2/1
  Product2/1 -> Sum9/2
  Sum9/1 -> ogr/1, V/1, Integrator/1
  Constant5/1 -> Генераці/1(In1)
  Sum4/1 -> Генераці/Trigger
  Генераці/1(Out1) -> Switch1/2
  Switch1/1 -> Sum8/1
  постійні/4(Out4) -> Sum4/1
  Constant1/1 -> Генераці1/1(In1)
  Sum1/1 -> Генераці1/Trigger
  Генераці1/1(Out1) -> Switch2/2
  Switch2/1 -> Sum8/2
  ogr/1 -> Out2/1
  Constant2/1 -> Генераці2/1(In1)
  Генераці2/1(Out1) -> Switch3/2
  Sum2/1 -> Генераці2/Trigger
  Sum8/1 -> Switch3/3
  Switch3/1 -> Out1/1, V1/1
  постійні/5(Out5) -> Sum1/1
  T-Загальний час циклу,с/1 -> Sum2/2
  Integrator/1 -> Product5/2
  Product5/1 -> Scope2/1, Out3/1
  Divide/1 -> Product5/1
  Constant/1 -> Divide/1

== system model_min_mine/5 систем підйому/3/4-періодна /Генераці ==
  In1 : Inport
  Trigger : TriggerPort  TriggerType=either  VariantControl=(inherit)  ShowOutputPort=on
  Out1 : Outport
  wires:
  In1/1 -> Out1/1

== system model_min_mine/5 систем підйому/3/4-періодна /Генераці1 ==
  In1 : Inport
  Trigger : TriggerPort  TriggerType=either  VariantControl=(inherit)  ShowOutputPort=on
  Out1 : Outport
  wires:
  In1/1 -> Out1/1

== system model_min_mine/5 систем підйому/3/4-періодна /Генераці2 ==
  In1 : Inport
  Trigger : TriggerPort  TriggerType=either  VariantControl=(inherit)  ShowOutputPort=on
  Out1 : Outport
  wires:
  In1/1 -> Out1/1

== system model_min_mine/5 систем підйому/3/4-періодна /Генераці3 ==
  In1 : Inport
  Trigger : TriggerPort  TriggerType=either  VariantControl=(inherit)  ShowOutputPort=on
  Out1 : Outport
  wires:
  In1/1 -> Out1/1

== system model_min_mine/5 систем підйому/3/4-періодна /постійні ==
  (t1) : Constant  Value=1.15
  (t3) : Constant  Value=2
  (t4) : Constant
  T : Constant  Value=7.15
  a1 : Constant  Value=0.5
  a3 : Constant  Value=-1
  a4 : Constant  Value=-0.95
  Out1 : Outport
  Out2 : Outport  Port=2
  Out6 : Outport  Port=3
  Out3 : Outport  Port=4
  Out4 : Outport  Port=5
  Out5 : Outport  Port=6
  Out7 : Outport  Port=7
  wires:
  a1/1 -> Out1/1
  a3/1 -> Out2/1
  (t3)/1 -> Out3/1
  (t1)/1 -> Out4/1
  (t4)/1 -> Out5/1
  a4/1 -> Out6/1
  T/1 -> Out7/1

== system model_min_mine/5 систем підйому/3/5-періодні/криво ==
  note: затримка на
      |  (t1)
  note: затримка на
      |  (t1+ t2 + t3)
  note: затримка на
      |  (t1+ t2 +t3 +t4)
  (t-2) : Saturate  UpperLimit=3.5  LowerLimit=0
  (t-4) : Saturate  UpperLimit=3.5  LowerLimit=0
  (t-5) : Saturate  LowerLimit=0
  (t1) : Saturate  LowerLimit=0
  Clock1 : Clock
      settings: Decimation=14
  Constant : Constant  Value=2
  Divide : Product  Inputs=/
  Integrator : Integrator
  Product{2..6} (5 alike) : Product  SaturateOnIntegerOverflow=on  OutDataTypeStr=Inherit: Same as first input
  Scope{1..3,5..7,9} (7 alike) : Scope
  Subsystem : Subsystem
  Subsystem1 : Subsystem
  Subsystem2 : Subsystem
  Subsystem3 : Subsystem
  Subsystem6 : Subsystem
  Sum1 : Sum  Inputs=|++++  SaturateOnIntegerOverflow=on
  Sum2 : Sum  Inputs=|++++  SaturateOnIntegerOverflow=on
  t1 : DeadZone  LowerValue=0  UpperValue=11.5  SaturateOnIntegerOverflow=on
  t2 : DeadZone  LowerValue=0  SaturateOnIntegerOverflow=on
  t5 : DeadZone  LowerValue=0  UpperValue=8  SaturateOnIntegerOverflow=on
  Допоміжний : Subsystem
  Допоміжний1 : Subsystem
  постійні : Subsystem
  Out1 : Outport
  Out2 : Outport  Port=2
  Out3 : Outport  Port=3
  wires:
  t2/1 -> (t-2)/1
  Clock1/1 -> t2/1, t5/1, t1/1, Subsystem6/2(t), Subsystem3/1(t1), Subsystem2/1(t1), (t1)/1
  постійні/5(Out5) -> Subsystem/1(t1)
  постійні/1(Out1) -> Product6/2, Subsystem/3(a1)
  (t-2)/1 -> Product4/1, Subsystem1/2(t)
  постійні/6(Out6) -> Subsystem1/1(t1)
  постійні/2(Out2) -> Product4/2, Subsystem1/3(a1)
  t5/1 -> (t-4)/1
  (t-4)/1 -> Product2/1, Допоміжний1/2(t)
  t1/1 -> (t-5)/1
  (t-5)/1 -> Product3/1
  постійні/3(Out3) -> Subsystem2/3(a1), Product2/2
  постійні/4(Out4) -> Subsystem3/3(a1), Product3/2
  Subsystem6/1(Out1) -> Out1/1, Scope1/1
  Product4/1 -> Sum1/2
  Product6/1 -> Sum1/1
  Sum1/1 -> Scope3/1, Out2/1, Integrator/1
  Subsystem/1(Out1) -> Допоміжний/1(t1), Scope5/1, Sum2/2
  (t1)/1 -> Product6/1, Subsystem/2(t), Допоміжний/2(t)
  Sum2/1 -> Subsystem6/3(a), Scope7/1
  постійні/9(Out9) -> Subsystem6/1(Сума t)
  Product2/1 -> Sum1/3, Scope6/1
  Product3/1 -> Sum1/4
  Subsystem3/1(Out1) -> Scope9/1, Sum2/4
  Subsystem1/1(Out1) -> Допоміжний/3(a1)
  Допоміжний/1(Out1) -> Sum2/1
  постійні/10(Out10) -> Subsystem2/2(t)
  Subsystem2/1(Out1) -> Допоміжний1/3(a1)
  Допоміжний1/1(Out1) -> Sum2/3
  постійні/7(Out7) -> Допоміжний1/1(t1)
  постійні/8(Out8) -> Subsystem3/2(t)
  Integrator/1 -> Product5/2
  Product5/1 -> Scope2/1, Out3/1
  Divide/1 -> Product5/1
  Constant/1 -> Divide/1

== system model_min_mine/5 систем підйому/3/5-періодні/пр ==
  note: затримка на
      |  (t1)
  note: затримка на
      |  (t1+ t2)
  note: затримка на
      |  (t1+ t2 +t3 +t4)
  note: затримка на
      |  (t1+ t2 +t3 +t4 +t5)
  note: затримка на
      |  (t1+ t2 +t3 +t4 +t5 + t6)
  (t-2) : Saturate  UpperLimit=3.5  LowerLimit=0
  (t-3) : Saturate  LowerLimit=0
  (t-5) : Saturate  LowerLimit=0
  (t-6) : Saturate  UpperLimit=3.5  LowerLimit=0
  (t-7) : Saturate  LowerLimit=0
  (t1) : Saturate  LowerLimit=0
  Clock1 : Clock
      settings: Decimation=14
  Constant : Constant  Value=2
  Divide : Product  Inputs=/
  Integrator : Integrator
  Product{1,4..7} (5 alike) : Product  SaturateOnIntegerOverflow=on  OutDataTypeStr=Inherit: Same as first input
  Scope{1..3,5} (4 alike) : Scope
  Subsystem : Subsystem
  Subsystem1 : Subsystem
  Subsystem4 : Subsystem
  Subsystem5 : Subsystem
  Subsystem6 : Subsystem
  Sum1 : Sum  Inputs=|++++++  SaturateOnIntegerOverflow=on
  Sum2 : Sum  Inputs=|++++  SaturateOnIntegerOverflow=on
  Sum3 : Sum  Inputs=-  SaturateOnIntegerOverflow=on
  t1 : DeadZone  LowerValue=0  UpperValue=7.5  SaturateOnIntegerOverflow=on
  t2 : DeadZone  LowerValue=0  SaturateOnIntegerOverflow=on
  t3 : DeadZone  LowerValue=0  UpperValue=8  SaturateOnIntegerOverflow=on
  t4 : DeadZone  LowerValue=0  UpperValue=11.5  SaturateOnIntegerOverflow=on
  t5 : DeadZone  LowerValue=0  UpperValue=4  SaturateOnIntegerOverflow=on
  Допоміжний : Subsystem
  Допоміжний -1 : Subsystem
  Допоміжний -2 : Subsystem
  Допоміжний -3 : Subsystem
  Допоміжний -4 : Subsystem
  пакет1 : Subsystem
  пакет2 : Subsystem
  постійні : Subsystem
  Out1 : Outport
  Out2 : Outport  Port=2
  Out3 : Outport  Port=3
  wires:
  t2/1 -> (t-2)/1
  Clock1/1 -> t2/1, t5/1, t1/1, t3/1, t4/1, Subsystem6/2(t), (t1)/1
  постійні/7(Out7) -> Subsystem/1(t1)
  постійні/1(Out1) -> Product6/2, Subsystem/3(a1)
  (t-2)/1 -> Product4/1, Subsystem1/2(t), Допоміжний -1/2(t)
  постійні/8(Out8) -> Subsystem1/1(t1)
  постійні/2(Out2) -> Product4/2, Subsystem1/3(a1)
  t5/1 -> (t-3)/1
  (t-3)/1 -> пакет1/2(t), Допоміжний -2/2(t)
  t1/1 -> (t-5)/1
  (t-5)/1 -> пакет2/2(t), Допоміжний -3/2(t)
  постійні/9(Out9) -> пакет1/1(ti)
  постійні/11(Out11) -> пакет2/1(ti)
  постійні/3(Out3) -> пакет1/3(a)
  постійні/4(Out4) -> пакет2/3(a)
  t3/1 -> (t-6)/1
  (t-6)/1 -> Product5/1, Subsystem4/2(t), Допоміжний -4/2(t)
  постійні/12(Out12) -> Subsystem4/1(ti)
  постійні/5(Out5) -> Subsystem4/3(a), Product5/2
  t4/1 -> (t-7)/1
  (t-7)/1 -> Subsystem5/2(t), Product7/1
  постійні/13(Out13) -> Subsystem5/1(ti)
  постійні/6(Out6) -> Product7/2, Subsystem5/3(a)
  постійні/10(Out10) -> Subsystem6/1(Сума t)
  Subsystem6/1(Out1) -> Out1/1, Scope1/1
  Product4/1 -> Sum1/2
  Product6/1 -> Sum1/1
  пакет1/2(Out2) -> Sum1/3
  пакет2/2(Out2) -> Sum1/4
  Product5/1 -> Sum1/5
  Product7/1 -> Sum1/6
  Sum1/1 -> Scope3/1, Out2/1, Integrator/1
  Subsystem/1(Out1) -> Допоміжний/1(t1), Sum2/2, Scope5/1
  (t1)/1 -> Product6/1, Subsystem/2(t), Допоміжний/2(t)
  Subsystem1/1(Out1) -> Допоміжний/3(a1)
  Допоміжний/1(Out1) -> Допоміжний -1/1(t1)
  пакет1/1(Out1) -> Допоміжний -1/3(a1)
  Допоміжний -1/1(Out1) -> Допоміжний -2/1(t1), Sum2/1
  пакет2/1(Out1) -> Допоміжний -2/3(a1)
  Допоміжний -2/1(Out1) -> Допоміжний -3/1(t1), Sum2/3
  Subsystem4/1(Out1) -> Допоміжний -3/3(a1)
  Допоміжний -3/1(Out1) -> Допоміжний -4/1(t1)
  Subsystem5/1(Out1) -> Допоміжний -4/3(a1)
  Sum2/1 -> Subsystem6/3(a)
  Допоміжний -4/1(Out1) -> Sum3/1
  Sum3/1 -> Sum2/4
  Integrator/1 -> Product1/2
  Product1/1 -> Scope2/1, Out3/1
  Divide/1 -> Product1/1
  Constant/1 -> Divide/1

== system model_min_mine/5 систем підйому/3/6-періодні/6-ти періодна криволінійна ==
  note: затримка на
      |  (t1)
  note: затримка на
      |  (t1+ t2 + t3)
  note: затримка на
      |  (t1+ t2 +t3 +t4 +t4/)
  (t-2) : Saturate  UpperLimit=3.5  LowerLimit=0
  (t-4) : Saturate  UpperLimit=3.5  LowerLimit=0
  (t-5) : Saturate  LowerLimit=0
  (t1) : Saturate  LowerLimit=0
  Clock1 : Clock
      settings: Decimation=14
  Constant : Constant  Value=2
  Divide : Product  Inputs=/
  Integrator : Integrator
  Product3 : Product  SaturateOnIntegerOverflow=on  OutDataTypeStr=Inherit: Same as first input
  Product5 : Product  SaturateOnIntegerOverflow=on  OutDataTypeStr=Inherit: Same as first input
  Product6 : Product  SaturateOnIntegerOverflow=on  OutDataTypeStr=Inherit: Same as first input
  Scope{1..3,5,7,9} (6 alike) : Scope
  Scope6 : Scope  NumInputPorts=3
  Subsystem : Subsystem
  Subsystem3 : Subsystem
  Subsystem6 : Subsystem
  Sum1 : Sum  Inputs=|++++  SaturateOnIntegerOverflow=on
  Sum2 : Sum  Inputs=|++++  SaturateOnIntegerOverflow=on
  t1 : DeadZone  LowerValue=0  UpperValue=12  SaturateOnIntegerOverflow=on
  t2 : DeadZone  LowerValue=0  SaturateOnIntegerOverflow=on
  t5 : DeadZone  LowerValue=0  UpperValue=8  SaturateOnIntegerOverflow=on
  Допоміжний : Subsystem
  Допоміжний1 : Subsystem
  пакет1 : Subsystem
  пакет2 : Subsystem
  постійні : Subsystem
  Out1 : Outport
  Out2 : Outport  Port=2
  Out3 : Outport  Port=3
  wires:
  t2/1 -> (t-2)/1
  Clock1/1 -> (t1)/1, t2/1, t5/1, t1/1, Subsystem6/2(t), Subsystem3/1(t1)
  постійні/5(Out5) -> Subsystem/1(t1)
  постійні/1(Out1) -> Product6/2, Subsystem/3(a1)
  (t-2)/1 -> пакет1/2(t)
  постійні/6(Out6) -> пакет1/1(ti)
  постійні/2(Out2) -> пакет1/3(a)
  t5/1 -> (t-4)/1
  (t-4)/1 -> Допоміжний1/2(t), пакет2/2(t)
  t1/1 -> (t-5)/1
  (t-5)/1 -> Product3/1
  постійні/3(Out3) -> пакет2/3(a)
  постійні/4(Out4) -> Subsystem3/3(a1), Product3/2
  Subsystem6/1(Out1) -> Out1/1, Scope1/1
  Product6/1 -> Sum1/1
  Sum1/1 -> Scope3/1, Out2/1, Scope6/2, Integrator/1
  Subsystem/1(Out1) -> Допоміжний/1(t1), Scope5/1, Sum2/2
  (t1)/1 -> Product6/1, Subsystem/2(t), Допоміжний/2(t)
  Sum2/1 -> Subsystem6/3(a), Scope7/1
  постійні/9(Out9) -> Subsystem6/1(Сума t)
  Product3/1 -> Sum1/4
  Subsystem3/1(Out1) -> Scope9/1, Sum2/4, Scope6/3
  пакет1/1(Out1) -> Допоміжний/3(a1)
  Допоміжний/1(Out1) -> Sum2/1
  пакет2/1(Out1) -> Допоміжний1/3(a1)
  Допоміжний1/1(Out1) -> Sum2/3, Scope6/1
  постійні/7(Out7) -> Допоміжний1/1(t1), пакет2/1(ti)
  постійні/8(Out8) -> Subsystem3/2(t)
  пакет1/2(Out2) -> Sum1/2
  пакет2/2(Out2) -> Sum1/3
  Integrator/1 -> Product5/2
  Product5/1 -> Scope2/1, Out3/1
  Divide/1 -> Product5/1
  Constant/1 -> Divide/1

== system model_min_mine/5 систем підйому/3/6-періодні/6-ти періодна пр ==
  note: затримка на
      |  (t1)
  note: затримка на
      |  (t1+ t2 + t3)
  note: затримка на
      |  (t1+ t2 +t3 +t4 +t4/)
  (t-2) : Saturate  UpperLimit=3.5  LowerLimit=0
  (t-4) : Saturate  UpperLimit=3.5  LowerLimit=0
  (t-5) : Saturate  LowerLimit=0
  (t1) : Saturate  LowerLimit=0
  Clock1 : Clock
      settings: Decimation=14
  Constant : Constant  Value=2
  Divide : Product  Inputs=/
  Integrator : Integrator
  Product{2..6} (5 alike) : Product  SaturateOnIntegerOverflow=on  OutDataTypeStr=Inherit: Same as first input
  Scope{1..3,5,7,9} (6 alike) : Scope
  Scope6 : Scope  NumInputPorts=3
  Subsystem : Subsystem
  Subsystem1 : Subsystem
  Subsystem2 : Subsystem
  Subsystem3 : Subsystem
  Subsystem6 : Subsystem
  Sum1 : Sum  Inputs=|++++  SaturateOnIntegerOverflow=on
  Sum2 : Sum  Inputs=|++++  SaturateOnIntegerOverflow=on
  t1 : DeadZone  LowerValue=0  UpperValue=12  SaturateOnIntegerOverflow=on
  t2 : DeadZone  LowerValue=0  SaturateOnIntegerOverflow=on
  t5 : DeadZone  LowerValue=0  UpperValue=8  SaturateOnIntegerOverflow=on
  Допоміжний : Subsystem
  Допоміжний1 : Subsystem
  постійні : Subsystem
  Out1 : Outport
  Out2 : Outport  Port=2
  Out3 : Outport  Port=3
  wires:
  t2/1 -> (t-2)/1
  Clock1/1 -> t2/1, t5/1, t1/1, Subsystem6/2(t), Subsystem3/1(t1), Subsystem2/1(t1), (t1)/1
  постійні/5(Out5) -> Subsystem/1(t1)
  постійні/1(Out1) -> Product6/2, Subsystem/3(a1)
  (t-2)/1 -> Product4/1, Subsystem1/2(t)
  постійні/6(Out6) -> Subsystem1/1(t1)
  постійні/2(Out2) -> Product4/2, Subsystem1/3(a1)
  t5/1 -> (t-4)/1
  (t-4)/1 -> Product2/1, Допоміжний1/2(t)
  t1/1 -> (t-5)/1
  (t-5)/1 -> Product3/1
  постійні/3(Out3) -> Subsystem2/3(a1), Product2/2
  постійні/4(Out4) -> Subsystem3/3(a1), Product3/2
  Subsystem6/1(Out1) -> Out1/1, Scope1/1
  Product4/1 -> Sum1/2
  Product6/1 -> Sum1/1
  Sum1/1 -> Scope3/1, Out2/1, Scope6/2, Integrator/1
  Subsystem/1(Out1) -> Допоміжний/1(t1), Scope5/1, Sum2/2
  (t1)/1 -> Product6/1, Subsystem/2(t), Допоміжний/2(t)
  Sum2/1 -> Subsystem6/3(a), Scope7/1
  постійні/9(Out9) -> Subsystem6/1(Сума t)
  Product2/1 -> Sum1/3
  Product3/1 -> Sum1/4
  Subsystem3/1(Out1) -> Scope9/1, Sum2/4, Scope6/3
  Subsystem1/1(Out1) -> Допоміжний/3(a1)
  Допоміжний/1(Out1) -> Sum2/1
  постійні/10(Out10) -> Subsystem2/2(t)
  Subsystem2/1(Out1) -> Допоміжний1/3(a1)
  Допоміжний1/1(Out1) -> Sum2/3, Scope6/1
  постійні/7(Out7) -> Допоміжний1/1(t1)
  постійні/8(Out8) -> Subsystem3/2(t)
  Integrator/1 -> Product5/2
  Product5/1 -> Scope2/1, Out3/1
  Divide/1 -> Product5/1
  Constant/1 -> Divide/1

== system model_min_mine/5 систем підйому/3/7-періодні/7-ми періодна криволінійна ==
  note: затримка на
      |  (t1+t1/)
  note: затримка на
      |  (t1+ t2 + t3)
  note: затримка на
      |  (t1+ t2 +t3 + t4 + t4/)
  (t-2) : Saturate  UpperLimit=3.5  LowerLimit=0
  (t-4) : Saturate  UpperLimit=3.5  LowerLimit=0
  (t-5) : Saturate  LowerLimit=0
  (t1) : Saturate  LowerLimit=0
  Clock1 : Clock
      settings: Decimation=14
  Constant : Constant  Value=2
  Divide : Product  Inputs=/
  Integrator : Integrator
  Product3 : Product  SaturateOnIntegerOverflow=on  OutDataTypeStr=Inherit: Same as first input
  Product5 : Product  SaturateOnIntegerOverflow=on  OutDataTypeStr=Inherit: Same as first input
  Product6 : Product  SaturateOnIntegerOverflow=on  OutDataTypeStr=Inherit: Same as first input
  Scope1 : Scope  NumInputPorts=2
  Scope{3..5,7..9} (6 alike) : Scope
  Scope6 : Scope  NumInputPorts=3
  Subsystem : Subsystem
  Subsystem3 : Subsystem
  Subsystem6 : Subsystem
  Sum1 : Sum  Inputs=|++++  SaturateOnIntegerOverflow=on
  Sum2 : Sum  Inputs=|++++  SaturateOnIntegerOverflow=on
  t1 : DeadZone  LowerValue=0  UpperValue=12  SaturateOnIntegerOverflow=on
  t2 : DeadZone  LowerValue=0  UpperValue=1  SaturateOnIntegerOverflow=on
  t5 : DeadZone  LowerValue=0  UpperValue=8  SaturateOnIntegerOverflow=on
  Допоміжний : Subsystem
  Допоміжний1 : Subsystem
  пакет1 : Subsystem
  пакет2 : Subsystem
  постійні : Subsystem
  Out1 : Outport
  Out2 : Outport  Port=2
  Out3 : Outport  Port=3
  wires:
  t2/1 -> (t-2)/1
  Clock1/1 -> t2/1, t5/1, t1/1, Subsystem6/2(t), Subsystem3/1(t1), (t1)/1, Допоміжний/2(t)
  постійні/5(Out5) -> Subsystem/1(t1)
  постійні/1(Out1) -> Product6/2, Subsystem/3(a1)
  (t-2)/1 -> пакет1/2(t)
  постійні/6(Out6) -> пакет1/1(ti)
  постійні/2(Out2) -> пакет1/3(a)
  t5/1 -> (t-4)/1
  (t-4)/1 -> Допоміжний1/2(t), пакет2/2(t)
  t1/1 -> (t-5)/1
  (t-5)/1 -> Product3/1
  постійні/3(Out3) -> пакет2/3(a)
  постійні/4(Out4) -> Subsystem3/3(a1), Product3/2
  Subsystem6/1(Out1) -> Out1/1, Scope1/1
  Product6/1 -> Sum1/1
  Sum1/1 -> Scope3/1, Out2/1, Scope6/2, Scope1/2, Integrator/1
  Subsystem/1(Out1) -> Sum2/2
  (t1)/1 -> Product6/1, Subsystem/2(t)
  Sum2/1 -> Subsystem6/3(a), Scope7/1
  постійні/9(Out9) -> Subsystem6/1(Сума t)
  Product3/1 -> Sum1/4
  Subsystem3/1(Out1) -> Scope9/1, Sum2/4, Scope6/3
  пакет1/1(Out1) -> Допоміжний/3(a1), Scope8/1
  Допоміжний/1(Out1) -> Sum2/1, Scope5/1
  пакет2/1(Out1) -> Допоміжний1/3(a1)
  Допоміжний1/1(Out1) -> Sum2/3, Scope6/1
  постійні/7(Out7) -> Допоміжний1/1(t1), пакет2/1(ti)
  постійні/8(Out8) -> Subsystem3/2(t)
  постійні/11(Out11) -> Допоміжний/1(t1)
  пакет1/2(Out2) -> Sum1/2
  пакет2/2(Out2) -> Sum1/3
  Integrator/1 -> Product5/2
  Product5/1 -> Scope4/1, Out3/1
  Divide/1 -> Product5/1
  Constant/1 -> Divide/1
